simulink model "H250_LOEUnknown_400HzHILV1"  (R2022a)
settings: Solver=FixedStepDiscrete  StartTime=0.0  StopTime=inf  FixedStep=Ts  RelTol=1e-3
InitFcn:
  | H250_LOEUnknown_400HzParam
values from neighbouring files (symbols this model uses):
  Ts = 1/400    (= 0.0025)    [H250HILConInit_400HzTypeXLOEUnknown.m]
libraries: pixhawk_slib_sensors_actuators x5, pixhawk_slib_uORB_RW x5, pixhawk_slib_misc_utils x1
settings Model: Creator=kcx06  LastModifiedBy=kcx06
settings SolverCC: AlgebraicLoopSolver=TrustRegion  PositivePriorityOrder=on  AutoInsertRateTranBlk=on
settings DataIOCC: SaveOutput=off  SignalLogging=off  DSMLogging=off  SaveTime=off  ReturnWorkspaceOutputs=off
settings OptimizationCC: DefaultParameterBehavior=Inlined  EnhancedBackFolding=on  PassReuseOutputArgsAs=Individual arguments  ZeroExternalMemoryAtStartup=off  ZeroInternalMemoryAtStartup=off  MaxStackSize=64  OptimizeBlockOrder=speed  DifferentSizesBufferReuse=on  OptimizationCustomize=off  EfficientTunableParamExpr=on
settings DebuggingCC: ParameterTunabilityLossMsg=error  UnconnectedInputMsg=warning  UnconnectedOutputMsg=warning  UnconnectedLineMsg=warning  SFMachineParentedDataDiag=warning
settings HardwareCC: ProdBitPerPointer=32  ProdBitPerSizeT=32  ProdBitPerPtrDiffT=32  ProdLargestAtomicInteger=Long  ProdLargestAtomicFloat=Double  ProdWordSize=32  ProdHWDeviceType=ARM Compatible->ARM Cortex
settings SFSimCC: MATLABDynamicMemAlloc=off
settings RTWCC: SystemTargetFile=ert.tlc  HardwareBoard=Pixhawk PX4  TLCOptions="-aInlineSetEventsForThisBaseRateFcn=TLC_FALSE -aSuppressMultiTaskScheduler=TLC_FALSE  -aRateBasedStepFcn=0"  TemplateMakefile=ert_default_tmf  GenerateReport=on  CustomSource=./px4_simulink_app_params.c  Toolchain=Pixhawk Toolchain  BuildConfiguration=Faster Runs  LaunchReport=on  DLArmComputeVersion=19.05
settings CodeAppCC: ForceParamTrailComments=on  IgnoreCustomStorageClasses=off  OperatorAnnotations=on  SimulinkDataObjDesc=on  SFDataObjDesc=on  InsertBlockDesc=on
settings ERTTargetCC: SupportComplex=off  SupportContinuousTime=on  InlinedParameterPlacement=NonHierarchical  ERTCustomFileTemplate=px4_codertarget_file_process.tlc

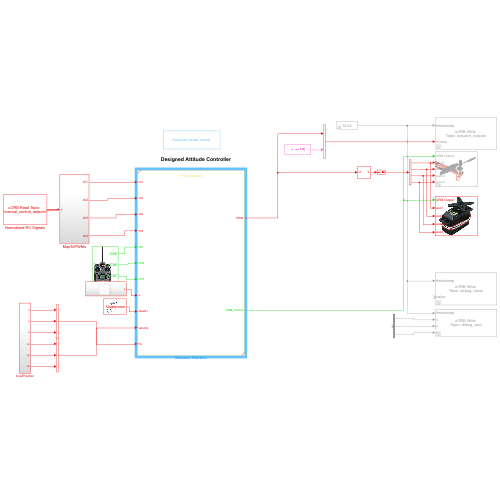
[thumbnail: Simulink's stored preview of the top-level diagram]
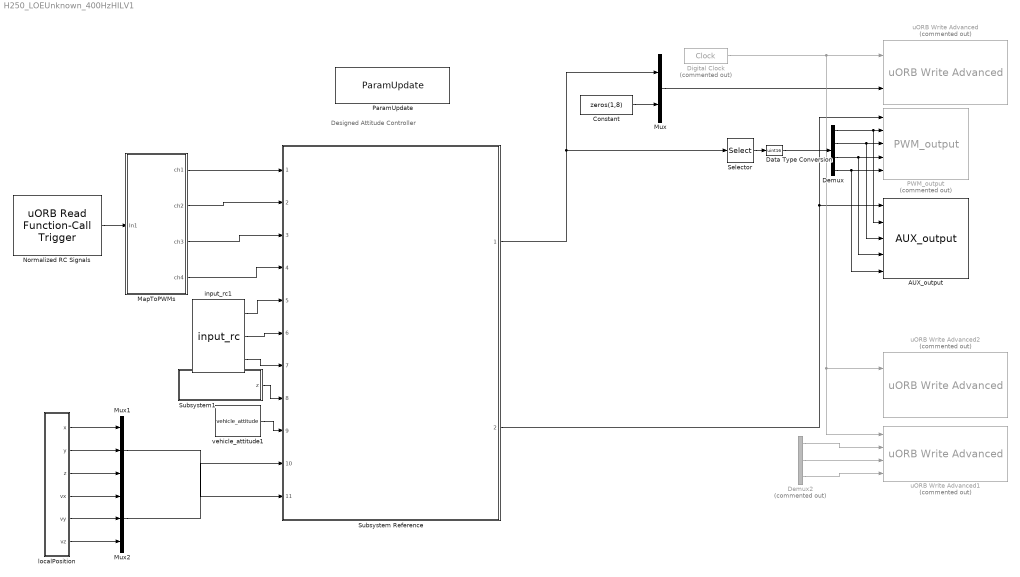
== system H250_LOEUnknown_400HzHILV1 ==
  note: Designed Attitude Controller
  AUX_output : pixhawk_slib_sensors_actuators/AUX_output  Description=|  pwm_rate=400Hz  show_aux1=on  show_aux4=on  show_aux2=on  show_aux5=off  show_aux3=on  show_aux6=off
      | This block allows the user to send the appropriate PWM signals out to the PX4 AUX outputs.  
      | These are usually connected to the ESCs which control the motor speeds. 
      | In order for the flight control to arm (enable) the output from the software side, the ARM Output input must be held high (boolean TRUE).  
      | Only then will the PWM values be sent out the PX4 hardware ports.  
      | This is usually a function of the RC Tx in combination with other flight modes programmed in the Simulink model by the user.  
      | The block has 8 available ports (data type uint16) which can be selectively chosen.  
      | These correspond to the 6 PWM (optional on 5/6) output ports on the px4fmu hardware. 
      | 
      | You *must* ensure that the line: “fmu mode_pwm” appears in your rc.txt file or manually run this from a Nuttx terminal *before* you start the px4_simulink_app module.  
      | Also – note: the FMU only has to be ARMED for the AUX pins to work – the Hardware safety switch is only for the IO.  
      | The switch’s blink code tells you what is armed.  You have to ARM both the Hardware switch and Software block in order to get the PWM output to work, but only the Software block for the AUX outputs.
      settings: SourceProductName=Pixhawk Target Blocks
  Constant : Constant  Value=zeros(1,8)  OutDataTypeStr=single
  Data Type Conversion : DataTypeConversion  OutDataTypeStr=uint16  SaturateOnIntegerOverflow=off  RndMeth=Floor
  Demux : Demux
  Demux2 : Demux  Commented=on  Outputs=3
  Digital Clock : DigitalClock  Commented=on  SampleTime=Ts
  MapToPWMs : Subsystem
  Mux : Mux  Inputs=2
  Mux1 : Mux  Inputs=3
  Mux2 : Mux  Inputs=3
  Normalized RC Signals : pixhawk_slib_uORB_RW/uORB Read Function-Call Trigger  uORB_Topic_str='manual_control_setpoint'  BusObjVar=Bus: manual_control_setpoint_SL  uORB_Interval=1  AsyncOutput=off  Fcn_call_select=Generate Function Call Signal  TaskName='Task1'  Poll_timeout=100  Ts=Ts
      settings: SourceProductName=Pixhawk Target Blocks
  PWM_output : pixhawk_slib_sensors_actuators/PWM_output  Description=|  Commented=on  pub_outputs=on  pwm_rate=400Hz  show_pwm1=on  show_pwm5=off  show_pwm2=on  show_pwm6=off  show_pwm3=on  show_pwm7=off  show_pwm4=on  show_pwm8=off
      | This block allows the user to send the appropriate PWM signals out to the PX4 outputs.  
      | These are usually connected to the ESCs which control the motor speeds. 
      | In order for the flight control to arm (enable) the output from the software side, the ARM Output input must be held high (boolean TRUE).  
      | Only then will the PWM values be sent out the PX4 hardware ports.  
      | This is usually a function of the RC Tx in combination with other flight modes programmed in the Simulink model by the user.  
      | The block has 8 available ports (data type uint16) which can be selectively chosen.  
      | These correspond to the 8 PWM output ports on the px4fmu hardware.
      settings: SourceProductName=Pixhawk Target Blocks
  ParamUpdate : pixhawk_slib_misc_utils/ParamUpdate  Description=|  Unformatted_StrSet=0  TLC_StrSet=0  NumParams=0  Ts=0
      | ParamUpdate Block
      | 
      | Use this block at your top-level of your model to insert a "parameter update" function in the generated code.
      settings: SourceProductName=Pixhawk Target Blocks
  Selector : Selector  IndexMode=Zero-based  InputPortWidth=8  IndexOptions=Index vector (dialog)  Indices=[0 1 2 3]  OutputSizes=1
  Subsystem Reference : Subsystem  ReferencedSubsystem=FTC_Unknown
  Subsystem1 : Subsystem
  input_rc1 : pixhawk_slib_sensors_actuators/input_rc  Description=|  sampletime=1/50  channel1=off  channel2=off  channel3=off  channel4=off  channel5=on  channel6=on  channel7=on  channel8=off  channel9=off  channel10=off  channel11=off  channel12=off  channel13=off  channel14=off  channel15=off  channel16=off  channel17=off  channel18=off  ch_count=off  rssi=off  rc_failsafe=off  rc_lost=off  rc_inputsource=off
      | RC Input Block
      | 
      | This block provides user input control to the model.
      | It uses the input_rc uORB topic.
      | 
      | The user has the ability to choose which channels are available as outputs from this block and also some optional outputs. These include 
      | Channels 1 through 18
      | double data type indicating the PWM value from the controller 
      | measured pulse widths for each of the supported channels 
      | Channel Count 
      | uint32 data type of the number of channels which are detector by the PX4 
      | RC Failsafe 
      | boolean data types indicating that the RC Tx is sending the FailSafe signal (if equipped and properly setup) 
      | explicit failsafe flag: true on TX failure or TX out of range , false otherwise. 
      | Only the true state is reliable, as there are some (PPM) receivers on the market going into failsafe without telling us explicitly. 
      | RC Input Source 
      | Enumeration data type indicating which source the RC input is from. 
      | Valid values are found in the ENUM file: RC_INPUT_SOURCE_ENUM.m 
      |           Enumeration members for class 'RC_INPUT_SOURCE_ENUM':
      |           RCINPUT_SOURCE_UNKNOWN         (0)
      |           RCINPUT_SOURCE_PX4FMU_PPM      (1)
      |           RCINPUT_SOURCE_PX4IO_PPM       (2)
      |           RCINPUT_SOURCE_PX4IO_SPEKTRUM  (3)
      |           RCINPUT_SOURCE_PX4IO_SBUS      (4)
      |           RCINPUT_SOURCE_PX4IO_ST24      (5)
      |           RCINPUT_SOURCE_MAVLINK         (6)
      |           RCINPUT_SOURCE_QURT            (7)
      |           RCINPUT_SOURCE_PX4FMU_SPEKTRUM (8)
      |           RCINPUT_SOURCE_PX4FMU_SBUS     (9)
      |           RCINPUT_SOURCE_PX4FMU_ST24     (10)
      |           RCINPUT_SOURCE_PX4FMU_SUMD     (11)
      |           RCINPUT_SOURCE_PX4FMU_DSM      (12)
      |           RCINPUT_SOURCE_PX4IO_SUMD      (13)
      | 
      | RSSI - Receive signal strength index 
      | receive signal strength indicator (RSSI): < 0: Undefined, 0: no signal, 255: full reception 
      | RC Lost Connection 
      | boolean data type indicating RC receiver connection status 
      | True, if no frame has arrived in the expected time, false otherwise. 
      | True usally means that the receiver has been disconnected, but can also indicate a radio link loss on "stupid" systems. 
      | Will remain false, if a RX with failsafe option continues to transmit frames after a link loss. 
      |   
      | Sample Model: px4demo_input_rc.slx
      settings: SourceProductName=Pixhawk Target Blocks
  "localPosition " : Subsystem
  uORB Write Advanced : pixhawk_slib_uORB_RW/uORB Write Advanced  Commented=on  Ts=0  uORB_AdvtQueue=on  uORB_FieldEnabledArr="0  0  0  1  0  0  0  0  0  0  0"  uORB_Topic_str=0  uORB_Struct_DT="[1  1  1  1  1]"  BlockInputCount=5  uORB_StructParams="[\"voltage_v\",\"voltage_filtered_v\",\"current_a\",\"current_filtered_a\",\"remaining\"]"  uORB_PortSizes="[1  1  1  1]"  MsgSizeOf=0  MW_update=true
      settings: SourceProductName=Pixhawk Target Blocks
  uORB Write Advanced1 : pixhawk_slib_uORB_RW/uORB Write Advanced  Commented=on  Ts=0  uORB_AdvtQueue=on  uORB_FieldEnabledArr="0  0  0  1  0  0  0  0  0  0  0"  uORB_Topic_str=0  uORB_Struct_DT="[1  1  1  1  1]"  BlockInputCount=5  uORB_StructParams="[\"voltage_v\",\"voltage_filtered_v\",\"current_a\",\"current_filtered_a\",\"remaining\"]"  uORB_PortSizes="[1  1  1  1]"  MsgSizeOf=0  MW_update=true
      settings: SourceProductName=Pixhawk Target Blocks
  uORB Write Advanced2 : pixhawk_slib_uORB_RW/uORB Write Advanced  Commented=on  Ts=0  uORB_AdvtQueue=on  uORB_FieldEnabledArr="0  0  0  1  0  0  0  0  0  0  0"  uORB_Topic_str=0  uORB_Struct_DT="[1  1  1  1  1]"  BlockInputCount=5  uORB_StructParams="[\"voltage_v\",\"voltage_filtered_v\",\"current_a\",\"current_filtered_a\",\"remaining\"]"  uORB_PortSizes="[1  1  1  1]"  MsgSizeOf=0  MW_update=true
      settings: SourceProductName=Pixhawk Target Blocks
  vehicle_attitude1 : pixhawk_slib_sensors_actuators/vehicle_attitude  sampletime=1/400  show_r=off  show_p=off  show_y=off  show_q=on  show_ts=off
      settings: SourceProductName=Pixhawk Target Blocks
  wires:
  Subsystem Reference/1 -> Selector/1, Mux/1
  Subsystem Reference/2 -> AUX_output/1, PWM_output/1
  MapToPWMs/4(ch4) -> Subsystem Reference/4
  Constant/1 -> Mux/2
  "localPosition "/5(vy) -> Mux2/2
  MapToPWMs/1(ch1) -> Subsystem Reference/1
  input_rc1/1 -> Subsystem Reference/5
  Mux1/1 -> Subsystem Reference/11
  "localPosition "/3(z) -> Mux1/3
  Mux2/1 -> Subsystem Reference/10
  "localPosition "/4(vx) -> Mux2/1
  MapToPWMs/3(ch3) -> Subsystem Reference/3
  "localPosition "/2(y) -> Mux1/2
  Normalized RC Signals/1 -> MapToPWMs/1(In1)
  Mux/1 -> uORB Write Advanced/2
  "localPosition "/1(x) -> Mux1/1
  MapToPWMs/2(ch2) -> Subsystem Reference/2
  Digital Clock/1 -> uORB Write Advanced1/1, uORB Write Advanced2/1, uORB Write Advanced/1
  "localPosition "/6(vz) -> Mux2/3
  input_rc1/2 -> Subsystem Reference/6
  vehicle_attitude1/1 -> Subsystem Reference/9
  Subsystem1/1(z) -> Subsystem Reference/8
  Selector/1 -> Data Type Conversion/1
  Demux/1 -> AUX_output/2, PWM_output/2
  Demux/2 -> PWM_output/3, AUX_output/3
  Demux/3 -> AUX_output/4, PWM_output/4
  Demux/4 -> AUX_output/5, PWM_output/5
  Data Type Conversion/1 -> Demux/1
  Demux2/3 -> uORB Write Advanced1/4
  Demux2/1 -> uORB Write Advanced1/2
  Demux2/2 -> uORB Write Advanced1/3
  input_rc1/3 -> Subsystem Reference/7

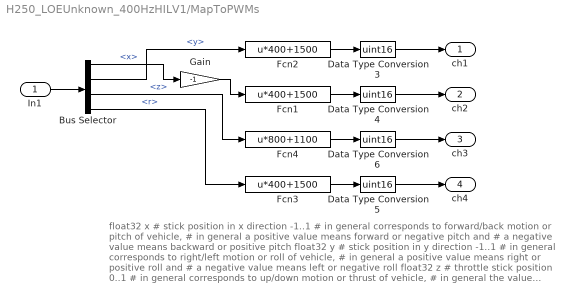
== system H250_LOEUnknown_400HzHILV1/MapToPWMs ==
  note: float32 x			 # stick position in x direction -1..1
      | 				 # in general corresponds to forward/back motion or pitch of vehicle,
      | 				 # in general a positive value means forward or negative pitch and
      | 				 # a negative value means backward or positive pitch
      | float32 y			 # stick position in y direction -1..1
      | 				 # in general corresponds to right/left motion or roll of vehicle,
      | 				 # in general a positive value means right or positive roll and
      | 				 # a negative value means left or negative roll
      | float32 z			 # throttle stick position 0..1
      | 				 # in general corresponds to up/down motion or thrust of vehicle,
      | 				 # in general the value corresponds to the demanded throttle by the user,
      | 				 # if the input is used for setting the setpoint of a vertical position
      | 				 # controller any value > 0.5 means up and any value < 0.5 means down
      | float32 r			 # yaw stick/twist position, -1..1
      | 				 # in general corresponds to the righthand rotation around the vertical
      | 				 # (downwards) axis of the vehicle
  In1 : Inport
  Bus Selector : BusSelector  OutputSignals=x,y,z,r
  Data Type Conversion{3..6} (4 alike) : DataTypeConversion  OutDataTypeStr=uint16  SaturateOnIntegerOverflow=off  RndMeth=Floor
  Fcn1 : Fcn  Expr=u*400+1500
  Fcn2 : Fcn  Expr=u*400+1500
  Fcn3 : Fcn  Expr=u*400+1500
  Fcn4 : Fcn  Expr=u*800+1100
  Gain : Gain  Gain=-1
  ch1 : Outport  VectorParamsAs1DForOutWhenUnconnected=off
  ch2 : Outport  Port=2  VectorParamsAs1DForOutWhenUnconnected=off
  ch3 : Outport  Port=3  VectorParamsAs1DForOutWhenUnconnected=off
  ch4 : Outport  Port=4  VectorParamsAs1DForOutWhenUnconnected=off
  wires:
  Bus Selector/2 -> Fcn2/1  "<y>"
  Fcn2/1 -> Data Type Conversion3/1
  Bus Selector/1 -> Gain/1  "<x>"
  In1/1 -> Bus Selector/1
  Bus Selector/3 -> Fcn4/1  "<z>"
  Fcn1/1 -> Data Type Conversion4/1
  Bus Selector/4 -> Fcn3/1  "<r>"
  Data Type Conversion4/1 -> ch2/1
  Data Type Conversion5/1 -> ch4/1
  Data Type Conversion6/1 -> ch3/1
  Fcn4/1 -> Data Type Conversion6/1
  Fcn3/1 -> Data Type Conversion5/1
  Data Type Conversion3/1 -> ch1/1
  Gain/1 -> Fcn1/1

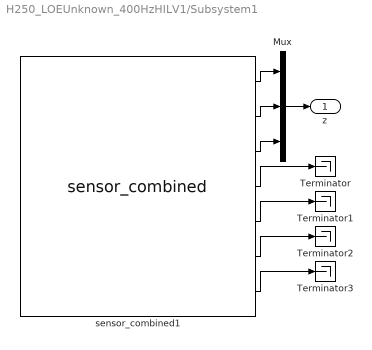
== system H250_LOEUnknown_400HzHILV1/Subsystem1 ==
  Mux : Mux  Inputs=3
  Terminator{,1..3} (4 alike) : Terminator
  sensor_combined1 : pixhawk_slib_sensors_actuators/sensor_combined  Description=|  sampletime=1/400  show_mag=off  show_acc=off  show_gyro=on  show_baro=off  show_ts=on
      | Sensor Combined Block
      | 
      | This block enables access to the various sensors available on the px4fmu-v2 hardware.  
      | The user can use these signals in the Simulink control model.  
      | The sample time needs to be provided in the mask dialog.  
      | Optional output ports can also be selected.  
      | Refer to the sample model: px4demo_attitude_control.slx
      | 
      | Signal definitions: 
      | Magnetometer (x,y,z) - single values – Magnetic field in NED body frame, in Gauss 
      | Accelerometer (x,y,z) - single values – Acceleration in NED body frame, in m/s^2 
      | Gyroscope (p,q,r) - single values – Angular velocity in radians per second 
      | Barometer (Altitude) - single value – Barometric pressure, already temperature compensated (millibars) 
      | RunTime (timestamp) - double value – Timestamp in microseconds since boot, from gyro 
      |   
      | The sensor_combined block needs to have the px4io service running on the PX4 hardware in order to get valid signal values.
      settings: SourceProductName=Pixhawk Target Blocks
  z : Outport
  wires:
  Mux/1 -> z/1
  sensor_combined1/1 -> Mux/1
  sensor_combined1/2 -> Mux/2
  sensor_combined1/3 -> Mux/3
  sensor_combined1/4 -> Terminator/1
  sensor_combined1/5 -> Terminator1/1
  sensor_combined1/6 -> Terminator2/1
  sensor_combined1/7 -> Terminator3/1

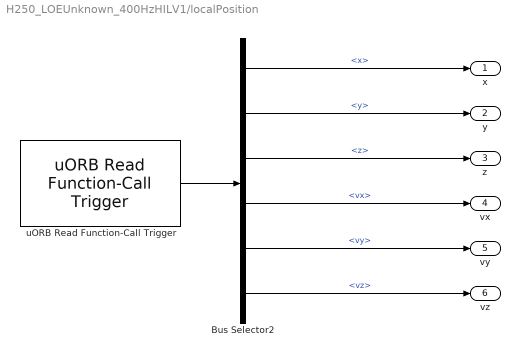
== system H250_LOEUnknown_400HzHILV1/localPosition  ==
  Bus Selector2 : BusSelector  OutputSignals=x,y,z,vx,vy,vz
  uORB Read Function-Call Trigger : pixhawk_slib_uORB_RW/uORB Read Function-Call Trigger  uORB_Topic_str='vehicle_local_position'  BusObjVar=Bus: vehicle_local_position_SL  uORB_Interval=1  AsyncOutput=off  Fcn_call_select=Generate Function Call Signal  TaskName='Task1'  Poll_timeout=100  Ts=Ts
      settings: SourceProductName=Pixhawk Target Blocks
  x : Outport  VectorParamsAs1DForOutWhenUnconnected=off
  y : Outport  Port=2  VectorParamsAs1DForOutWhenUnconnected=off
  z : Outport  Port=3  VectorParamsAs1DForOutWhenUnconnected=off
  vx : Outport  Port=4  VectorParamsAs1DForOutWhenUnconnected=off
  vy : Outport  Port=5  VectorParamsAs1DForOutWhenUnconnected=off
  vz : Outport  Port=6  VectorParamsAs1DForOutWhenUnconnected=off
  wires:
  uORB Read Function-Call Trigger/1 -> Bus Selector2/1
  Bus Selector2/1 -> x/1  "<x>"
  Bus Selector2/2 -> y/1  "<y>"
  Bus Selector2/3 -> z/1  "<z>"
  Bus Selector2/4 -> vx/1  "<vx>"
  Bus Selector2/5 -> vy/1  "<vy>"
  Bus Selector2/6 -> vz/1  "<vz>"
